simulink model "ProyectoGlobal_AyCD_Cantu_LagoTejo_OPCUA"  (R2021a)
settings: Solver=ode23  StartTime=0.0  StopTime=inf  MinStep=1e-4
undefined symbols (not defined in the file): a_hMax, a_tMax, b_cx, b_cy, b_eq_h, b_eq_t, b_hb, b_hEb, b_t, b_tb, b_tw, b_wu, bah, bat, bcx, bcy, CI_h, CI_t, Cond_Ini_h, Cond_Ini_t, g, H_c, i_h, i_t, k_cy, k_tw, k_wu, Kcy, Kd_bal, Kp_bal, ksah, ksat, ksiah, ksiat, lim_xDer, lim_xDer_ult, lim_xIzq, lim_xIzq_ult, lim_yInf, lim_yInf_ult, lim_ySup, lim_ySup_ult, M_cMax, M_cMin, M_eq_h, M_eq_t, M_s, M_t, r_hd, r_td, T_hbMax, T_hEbMax, T_hmMax, T_tbMax, T_tmMax, tau_hm, tau_tm, v_hMax_0, v_tMax, xc ... (+2)
libraries: simulink x13, opclib x3
(part 2 of 3)

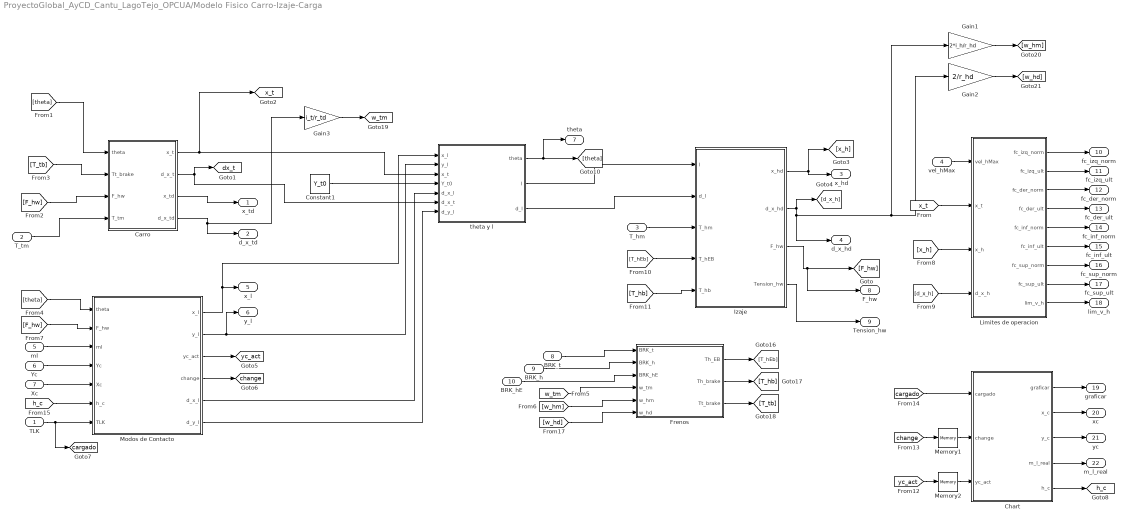
== system ProyectoGlobal_AyCD_Cantu_LagoTejo_OPCUA/Modelo Fisico Carro-Izaje-Carga ==
  TLK : Inport
  T_tm : Inport  Port=2
  T_hm : Inport  Port=3
  vel_hMax : Inport  Port=4
  ml : Inport  Port=5
  Yc : Inport  Port=6
  Xc : Inport  Port=7
  BRK_t : Inport  Port=8
  BRK_h : Inport  Port=9
  BRK_hE : Inport  Port=10
  Carro : Subsystem
  Chart : Stateflow chart  TreatAsAtomicUnit=on
      settings: PortSchema="{\"entries\":[{\"content\":{\"sides\":[{\"content\":{\"connectorIds\":[\"In1\",\"In2\",\"In3\"]},\"type\":\"ConnectorPlacement.EquallySpacedRectSide\",\"uuid\":\"3e82a7c2-bf75-4f61-8ed8-4dc94ac63b2a\"},{\"content\":{\"connectorIds\":[\"Out3\",\"Out4\",\"Out2\",\"Out5\",\"Out1\"],\"side\":\"RIGHT\"},\"type\":\"ConnectorPlacement.EquallySpacedRectSide\",\"uuid\":\"3bda0d7b-f5b8-4b7e-98a5-641e146bfa09\"},{\"content\":{\"connectorIds\":[],\"side\":\"TOP\"},\"type\":\"ConnectorPlacement.EquallySpacedRectSide\",\"uuid\":\"53c96370-adb7-4c5f-b84b-b565cd95f057\"}]},\"type\":\"ConnectorPlacement.EquallySpacedConnector\",\"uuid\":\"5926f053-77e4-4d2a-97aa-9f275575c8db\"}],\"packageUris\":[\"http://schema.mathworks.com/mf0/Connector/R2020b\"],\"version\":\"1.0\"}"
  Constant1 : Constant  Value=Y_t0
  Frenos : Subsystem
  Gain1 : Gain  Gain=2*i_h/r_hd
  Gain2 : Gain  Gain=2/r_hd
  Gain3 : Gain  Gain=i_t/r_td
  Izaje : Subsystem
  Limites de operacion : Subsystem
  Memory1 : Memory
  Memory2 : Memory
  Modos de Contacto : Subsystem
  theta y l : Subsystem
  x_td : Outport
  d_x_td : Outport  Port=2
  x_hd : Outport  Port=3
  d_x_hd : Outport  Port=4
  x_l : Outport  Port=5
  y_l : Outport  Port=6
  theta : Outport  Port=7
  F_hw : Outport  Port=8
  Tension_hw : Outport  Port=9
  fc_izq_norm : Outport  Port=10
  fc_izq_ult : Outport  Port=11
  fc_der_norm : Outport  Port=12
  fc_der_ult : Outport  Port=13
  fc_inf_norm : Outport  Port=14
  fc_inf_ult : Outport  Port=15
  fc_sup_norm : Outport  Port=16
  fc_sup_ult : Outport  Port=17
  lim_v_h : Outport  Port=18
  graficar : Outport  Port=19
  xc : Outport  Port=20
  yc : Outport  Port=21
  m_l_real : Outport  Port=22
  tag scope: cargado=global, change=global, dx_t=global, h_c=global, w_tm=global, x_t=global, yc_act=global
  wires:
  BRK_h/1 -> Frenos/2(BRK_h)
  BRK_t/1 -> Frenos/1(BRK_t)
  BRK_hE/1 -> Frenos/3(BRK_hE)
  [w_tm] -> Frenos/4(w_tm)
  [w_hm] -> Frenos/5(w_hm)
  Limites de operacion/2(fc_izq_ult) -> fc_izq_ult/1
  Limites de operacion/1(fc_izq_norm) -> fc_izq_norm/1
  Limites de operacion/6(fc_inf_ult) -> fc_inf_ult/1
  Gain2/1 -> [w_hd]
  Limites de operacion/9(lim_v_h) -> lim_v_h/1
  Limites de operacion/3(fc_der_norm) -> fc_der_norm/1
  Limites de operacion/4(fc_der_ult) -> fc_der_ult/1
  Limites de operacion/5(fc_inf_norm) -> fc_inf_norm/1
  Limites de operacion/7(fc_sup_norm) -> fc_sup_norm/1
  Gain3/1 -> [w_tm]
  vel_hMax/1 -> Limites de operacion/1(vel_hMax)
  Limites de operacion/8(fc_sup_ult) -> fc_sup_ult/1
  Gain1/1 -> [w_hm]
  Frenos/1(Th_EB) -> [T_hEb]
  Frenos/2(Th_brake) -> [T_hb]
  Frenos/3(Tt_brake) -> [T_tb]
  [w_hd] -> Frenos/6(w_hd)
  [theta] -> Carro/1(theta)
  [T_tb] -> Carro/2(Tt_brake)
  [F_hw] -> Carro/3(F_hw)
  T_tm/1 -> Carro/4(T_tm)
  Carro/2(d_x_t) -> theta y l/6(d_x_t), [dx_t]
  Carro/3(x_td) -> x_td/1
  Carro/4(d_x_td) -> Gain3/1, d_x_td/1
  Modos de Contacto/1(x_l) -> x_l/1, theta y l/1(x_l)
  Carro/1(x_t) -> [x_t], theta y l/3(x_t)
  Modos de Contacto/2(y_l) -> y_l/1, theta y l/2(y_l)
  theta y l/1(theta) -> [theta], theta/1
  Constant1/1 -> theta y l/4(Y_t0)
  Modos de Contacto/5(d_x_l) -> theta y l/5(d_x_l)
  Modos de Contacto/6(d_y_l) -> theta y l/7(d_y_l)
  [theta] -> Modos de Contacto/1(theta)
  [F_hw] -> Modos de Contacto/2(F_hw)
  ml/1 -> Modos de Contacto/3(ml)
  [h_c] -> Modos de Contacto/6(h_c)
  Yc/1 -> Modos de Contacto/4(Yc)
  Xc/1 -> Modos de Contacto/5(Xc)
  Modos de Contacto/4(change) -> [change]
  [T_hEb] -> Izaje/4(T_hEB)
  T_hm/1 -> Izaje/3(T_hm)
  [T_hb] -> Izaje/5(T_hb)
  theta y l/2(l) -> Izaje/1(l)
  theta y l/3(d_l) -> Izaje/2(d_l)
  Izaje/3(F_hw) -> F_hw/1, [F_hw]
  Izaje/1(x_hd) -> x_hd/1, [x_h]
  Izaje/2(d_x_hd) -> d_x_hd/1, Gain2/1, Gain1/1, [d_x_h]
  [x_t] -> Limites de operacion/2(x_t)
  [x_h] -> Limites de operacion/3(x_h)
  [d_x_h] -> Limites de operacion/4(d_x_h)
  Izaje/4(Tension_hw) -> Tension_hw/1
  [change] -> Memory1/1
  Chart/1(h_c) -> [h_c]
  Chart/4(x_c) -> xc/1
  Chart/3(graficar) -> graficar/1
  Chart/2(y_c) -> yc/1
  [yc_act] -> Memory2/1
  Modos de Contacto/3(yc_act) -> [yc_act]
  TLK/1 -> [cargado], Modos de Contacto/7(TLK)
  [cargado] -> Chart/1(cargado)
  Memory1/1 -> Chart/2(change)
  Memory2/1 -> Chart/3(yc_act)
  Chart/5(m_l_real) -> m_l_real/1

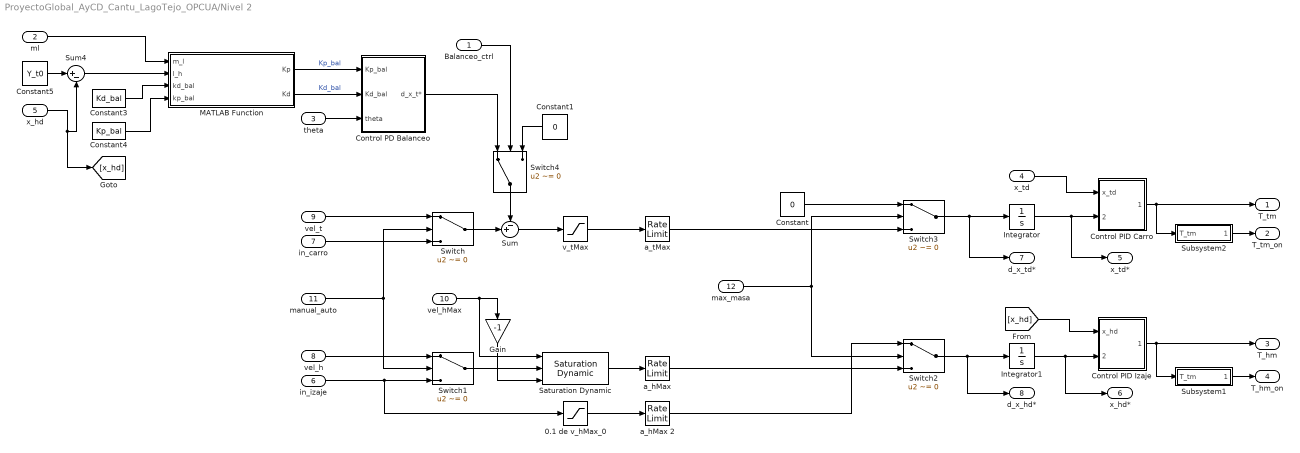
== system ProyectoGlobal_AyCD_Cantu_LagoTejo_OPCUA/Nivel 2 ==
  Balanceo_ctrl : Inport
  ml : Inport  Port=2
  theta : Inport  Port=3
  x_td : Inport  Port=4
  x_hd : Inport  Port=5
  in_izaje : Inport  Port=6
  in_carro : Inport  Port=7
  vel_h : Inport  Port=8
  vel_t : Inport  Port=9
  vel_hMax : Inport  Port=10
  manual_auto : Inport  Port=11
  max_masa : Inport  Port=12
  0.1 de v_hMax_0 : Saturate  UpperLimit=0  LowerLimit=-0.1*v_hMax_0
  Constant : Constant  Value=0
  Constant1 : Constant  Value=0
  Constant3 : Constant  Value=Kd_bal
  Constant4 : Constant  Value=Kp_bal
  Constant5 : Constant  Value=Y_t0
  Control PD Balanceo : Subsystem
  Control PID Carro : Subsystem
  Control PID Izaje : Subsystem
  Gain : Gain  Gain=-1
  Integrator : Integrator  InitialCondition=CI_t
  Integrator1 : Integrator  InitialCondition=CI_h
  MATLAB Function : MATLAB Function  TreatAsAtomicUnit=on
  Saturation Dynamic : simulink/Discontinuities/Saturation Dynamic  OutMin=[]  OutMax=[]  OutDataTypeStr=Inherit: Same as second input  OutDataType=fixdt(1, 16)  OutScaling=2^-10  DoSatur=off
  Subsystem1 : Subsystem
  Subsystem2 : Subsystem
  Sum : Sum  Inputs=-+|
  Sum4 : Sum  Inputs=|+-
  Switch{,1..4} (5 alike) : Switch  Criteria=u2 ~= 0
  a_hMax : RateLimiter  RisingSlewLimit=a_hMax  FallingSlewLimit=-a_hMax  SampleTimeMode=inherited
  a_hMax 2 : RateLimiter  RisingSlewLimit=a_hMax  FallingSlewLimit=-a_hMax  SampleTimeMode=inherited
  a_tMax : RateLimiter  RisingSlewLimit=a_tMax  FallingSlewLimit=-a_tMax  SampleTimeMode=inherited
  v_tMax : Saturate  UpperLimit=v_tMax  LowerLimit=-v_tMax
  T_tm : Outport
  T_tm_on : Outport  Port=2
  T_hm : Outport  Port=3
  T_hm_on : Outport  Port=4
  x_td* : Outport  Port=5
  x_hd* : Outport  Port=6
  d_x_td* : Outport  Port=7
  d_x_hd* : Outport  Port=8
  wires:
  manual_auto/1 -> Switch/2, Switch1/2
  Switch1/1 -> Saturation Dynamic/2
  vel_hMax/1 -> Saturation Dynamic/1, Gain/1
  Gain/1 -> Saturation Dynamic/3
  in_carro/1 -> Switch/3
  vel_h/1 -> Switch1/1
  Saturation Dynamic/1 -> a_hMax/1
  v_tMax/1 -> a_tMax/1
  Constant/1 -> Switch3/1
  0.1 de v_hMax_0/1 -> a_hMax 2/1
  vel_t/1 -> Switch/1
  Switch/1 -> Sum/2
  in_izaje/1 -> 0.1 de v_hMax_0/1, Switch1/3
  max_masa/1 -> Switch2/2, Switch3/2
  a_hMax 2/1 -> Switch2/1
  Sum/1 -> v_tMax/1
  a_tMax/1 -> Switch3/3
  a_hMax/1 -> Switch2/3
  Constant3/1 -> MATLAB Function/3(kd_bal)
  Balanceo_ctrl/1 -> Switch4/2
  Constant4/1 -> MATLAB Function/4(kp_bal)
  Constant5/1 -> Sum4/1
  x_hd/1 -> [x_hd], Sum4/2
  Sum4/1 -> MATLAB Function/2(l_h)
  ml/1 -> MATLAB Function/1(m_l)
  Constant1/1 -> Switch4/3
  MATLAB Function/1(Kp) -> Control PD Balanceo/1(Kp_bal)  "Kp_bal"
  MATLAB Function/2(Kd) -> Control PD Balanceo/2(Kd_bal)  "Kd_bal"
  theta/1 -> Control PD Balanceo/3(theta)
  Control PD Balanceo/1(d_x_t*) -> Switch4/1
  Switch4/1 -> Sum/1
  x_td/1 -> Control PID Carro/1(x_td)
  Integrator1/1 -> x_hd*/1, Control PID Izaje/2(x_hd*)
  [x_hd] -> Control PID Izaje/1(x_hd)
  Switch2/1 -> d_x_hd*/1, Integrator1/1
  Control PID Carro/1(T_tm) -> Subsystem2/1(T_tm), T_tm/1
  Integrator/1 -> x_td*/1, Control PID Carro/2(x_td*)
  Switch3/1 -> d_x_td*/1, Integrator/1
  Control PID Izaje/1(T_hm) -> T_hm/1, Subsystem1/1(T_tm)
  Subsystem1/1(T_tm_on) -> T_hm_on/1
  Subsystem2/1(T_tm_on) -> T_tm_on/1

== system ProyectoGlobal_AyCD_Cantu_LagoTejo_OPCUA/Subsystem ==
  " " : Inport
  AND : Logic  IconShape=distinctive  AllPortsSameDT=off  OutDataTypeStr=boolean
  BTN_RESET_PRESSED : Constant  Value=0
  Out1 : Outport
  wires:
  BTN_RESET_PRESSED/1 -> AND/2
  " "/1 -> AND/1
  AND/1 -> Out1/1

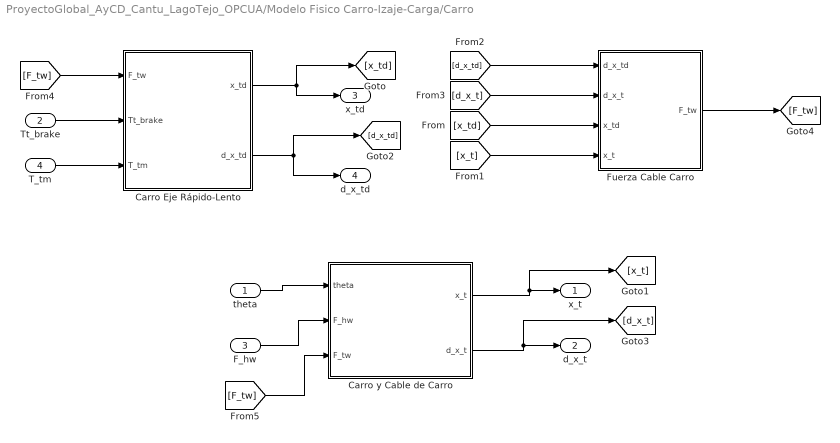
== system ProyectoGlobal_AyCD_Cantu_LagoTejo_OPCUA/Modelo Fisico Carro-Izaje-Carga/Carro ==
  theta : Inport
  Tt_brake : Inport  Port=2
  F_hw : Inport  Port=3
  T_tm : Inport  Port=4
  Carro Eje Rápido-Lento : Subsystem
  Carro y Cable de Carro : Subsystem
  Fuerza Cable Carro : Subsystem
  x_t : Outport
  d_x_t : Outport  Port=2
  x_td : Outport  Port=3
  d_x_td : Outport  Port=4
  wires:
  Tt_brake/1 -> Carro Eje Rápido-Lento/2(Tt_brake)
  theta/1 -> Carro y Cable de Carro/1(theta)
  Carro Eje Rápido-Lento/1(x_td) -> x_td/1, [x_td]
  Carro y Cable de Carro/2(d_x_t) -> [d_x_t], d_x_t/1
  Carro Eje Rápido-Lento/2(d_x_td) -> [d_x_td], d_x_td/1
  F_hw/1 -> Carro y Cable de Carro/2(F_hw)
  Carro y Cable de Carro/1(x_t) -> [x_t], x_t/1
  T_tm/1 -> Carro Eje Rápido-Lento/3(T_tm)
  [x_td] -> Fuerza Cable Carro/3(x_td)
  [x_t] -> Fuerza Cable Carro/4(x_t)
  Fuerza Cable Carro/1(F_tw) -> [F_tw]
  [d_x_td] -> Fuerza Cable Carro/1(d_x_td)
  [d_x_t] -> Fuerza Cable Carro/2(d_x_t)
  [F_tw] -> Carro Eje Rápido-Lento/1(F_tw)
  [F_tw] -> Carro y Cable de Carro/3(F_tw)

== system ProyectoGlobal_AyCD_Cantu_LagoTejo_OPCUA/Modelo Fisico Carro-Izaje-Carga/Frenos ==
  BRK_t : Inport
  BRK_h : Inport  Port=2
  BRK_hE : Inport  Port=3
  w_tm : Inport  Port=4
  w_hm : Inport  Port=5
  w_hd : Inport  Port=6
  Freno Emergencia Izaje : Subsystem
  Freno Operacion Carro : Subsystem
  Freno Operacion Izaje : Subsystem
  Th_EB : Outport
  Th_brake : Outport  Port=2
  Tt_brake : Outport  Port=3
  wires:
  Freno Operacion Izaje/1(Thb) -> Th_brake/1
  BRK_h/1 -> Freno Operacion Izaje/1(Energizado/Desenergizado)
  BRK_t/1 -> Freno Operacion Carro/1(Energizado/Desenergizado)
  Freno Operacion Carro/1(Ttb) -> Tt_brake/1
  BRK_hE/1 -> Freno Emergencia Izaje/1(Energizado/Desenergizado)
  Freno Emergencia Izaje/1(Th_EB) -> Th_EB/1
  w_tm/1 -> Freno Operacion Carro/2(w_tm)
  w_hm/1 -> Freno Operacion Izaje/2(w_hm)
  w_hd/1 -> Freno Emergencia Izaje/2(w_hd)

== system ProyectoGlobal_AyCD_Cantu_LagoTejo_OPCUA/Modelo Fisico Carro-Izaje-Carga/Izaje ==
  l : Inport
  d_l : Inport  Port=2
  T_hm : Inport  Port=3
  T_hEB : Inport  Port=4
  T_hb : Inport  Port=5
  Fuerza cable de Izaje : Subsystem
  Izaje Eje Rapido-Lento : Subsystem
  x_hd : Outport
  d_x_hd : Outport  Port=2
  F_hw : Outport  Port=3
  Tension_hw : Outport  Port=4
  wires:
  T_hb/1 -> Izaje Eje Rapido-Lento/4(T_hb)
  T_hEB/1 -> Izaje Eje Rapido-Lento/3(T_hEb)
  [F_hw] -> Izaje Eje Rapido-Lento/1(F_hw)
  T_hm/1 -> Izaje Eje Rapido-Lento/2(T_hm)
  Fuerza cable de Izaje/1(F_hw) -> [F_hw], F_hw/1
  d_l/1 -> Fuerza cable de Izaje/3(d_l)
  Izaje Eje Rapido-Lento/1(l_h) -> [l_h]
  Izaje Eje Rapido-Lento/3(x_hd) -> x_hd/1
  l/1 -> Fuerza cable de Izaje/1(l)
  Izaje Eje Rapido-Lento/4(d_x_hd) -> d_x_hd/1
  [l_h] -> Fuerza cable de Izaje/2(l_h)
  Izaje Eje Rapido-Lento/2(d_l_h) -> [d_l_h]
  [d_l_h] -> Fuerza cable de Izaje/4(d_l_h)
  Fuerza cable de Izaje/2(Tension_hw) -> Tension_hw/1

== system ProyectoGlobal_AyCD_Cantu_LagoTejo_OPCUA/Modelo Fisico Carro-Izaje-Carga/Limites de operacion ==
  vel_hMax : Inport
  x_t : Inport  Port=2
  x_h : Inport  Port=3
  d_x_h : Inport  Port=4
  Límites de Carro : Subsystem
  Subsystem1 : Subsystem
  fc_izq_norm : Outport
  fc_izq_ult : Outport  Port=2
  fc_der_norm : Outport  Port=3
  fc_der_ult : Outport  Port=4
  fc_inf_norm : Outport  Port=5
  fc_inf_ult : Outport  Port=6
  fc_sup_norm : Outport  Port=7
  fc_sup_ult : Outport  Port=8
  lim_v_h : Outport  Port=9
  wires:
  x_t/1 -> Límites de Carro/1(x_t)
  Límites de Carro/1(fc_izq_norm) -> fc_izq_norm/1
  Límites de Carro/2(fc_izq_ult) -> fc_izq_ult/1
  Límites de Carro/3(fc_der_norm) -> fc_der_norm/1
  Límites de Carro/4(fc_der_ult) -> fc_der_ult/1
  Subsystem1/4(fc_sup_ult) -> fc_sup_ult/1
  Subsystem1/3(fc_sup_norm) -> fc_sup_norm/1
  Subsystem1/2(fc_inf_ult) -> fc_inf_ult/1
  Subsystem1/1(fc_inf_norm) -> fc_inf_norm/1
  x_h/1 -> Subsystem1/1(x_h)
  d_x_h/1 -> Subsystem1/3(d_x_h)
  Subsystem1/5(lim_v_h) -> lim_v_h/1
  vel_hMax/1 -> Subsystem1/2(vel_hMax)

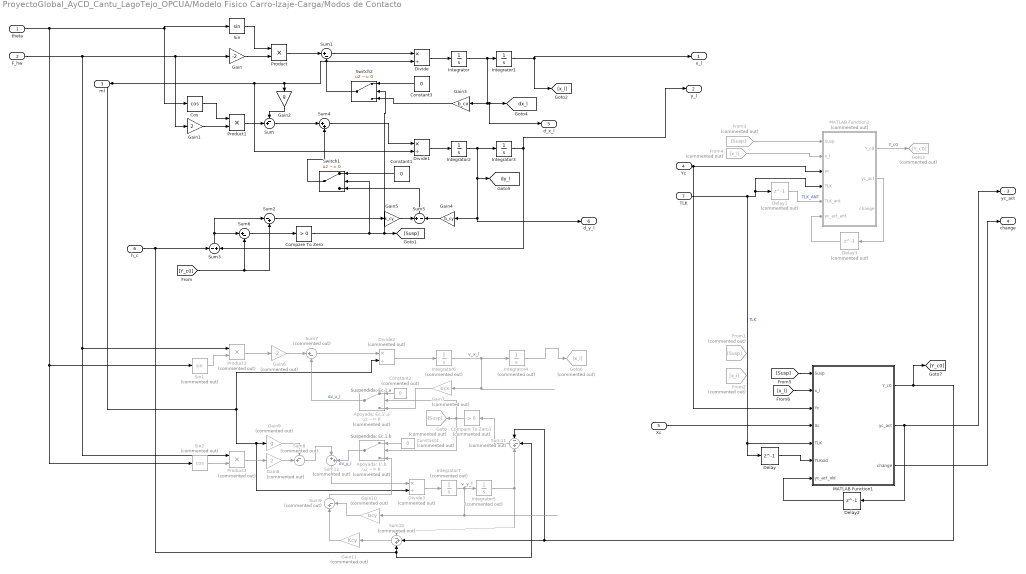
== system ProyectoGlobal_AyCD_Cantu_LagoTejo_OPCUA/Modelo Fisico Carro-Izaje-Carga/Modos de Contacto ==
  note: v_y_l
  note: v_x_l
  note: Suspendida: Ec.1.a
  note: Suspendida: Ec.1.b
  theta : Inport
  F_hw : Inport  Port=2
  ml : Inport  Port=3
  Yc : Inport  Port=4
  Xc : Inport  Port=5
  h_c : Inport  Port=6
  TLK : Inport  Port=7
  Apoyada: 1'.b : Switch  Commented=on  Criteria=u2 ~= 0
  Apoyada: Ec.1'.a : Switch  Commented=on  Criteria=u2 ~= 0
  Compare To Zero : simulink/Logic and Bit Operations/Compare To Zero  relop=>  OutDataTypeStr=boolean
  Compare To Zero1 : simulink/Logic and Bit Operations/Compare To Zero  Commented=on  relop=>  OutDataTypeStr=boolean
  Constant1 : Constant  Value=0
  Constant2 : Constant  Commented=on  Value=0
  Constant3 : Constant  Value=0
  Constant4 : Constant  Commented=on  Value=0
  Cos : Trigonometry  Operator=cos
  Delay : Delay  DelayLength=1
  Delay1 : Delay  Commented=on  DelayLength=1
  Delay2 : Delay  DelayLength=1
  Delay3 : Delay  Commented=on  DelayLength=1
  Divide : Product  Inputs=*/
  Divide1 : Product  Inputs=*/
  Divide2 : Product  Commented=on  Inputs=*/
  Divide3 : Product  Commented=on  Inputs=*/
  From1 : From  Commented=on  GotoTag=Susp
  From2 : From  Commented=on  GotoTag=x_l
  From3 : From  Commented=on  GotoTag=Susp
  From4 : From  Commented=on  GotoTag=x_l
  Gain : Gain  Gain=-2
  Gain1 : Gain  Gain=2
  Gain10 : Gain  Commented=on  Gain=bcy
  Gain11 : Gain  Commented=on  Gain=Kcy
  Gain2 : Gain  Gain=g
  Gain3 : Gain  Gain=b_cx
  Gain4 : Gain  Gain=b_cy
  Gain5 : Gain  Gain=k_cy
  Gain6 : Gain  Commented=on  Gain=-2
  Gain7 : Gain  Commented=on  Gain=bcx
  Gain8 : Gain  Commented=on  Gain=2
  Gain9 : Gain  Commented=on  Gain=g
  Goto : Goto  Commented=on  GotoTag=Susp
  Goto3 : Goto  Commented=on  GotoTag=Y_c0
  Goto6 : Goto  Commented=on  GotoTag=x_l
  Integrator : Integrator
  Integrator1 : Integrator  InitialCondition=CI_t
  Integrator2 : Integrator
  Integrator3 : Integrator  InitialCondition=CI_h
  Integrator4 : Integrator  Commented=on  InitialCondition=Cond_Ini_t
  Integrator5 : Integrator  Commented=on  InitialCondition=Cond_Ini_h
  Integrator6 : Integrator  Commented=on
  Integrator7 : Integrator  Commented=on
  MATLAB Function1 : MATLAB Function  TreatAsAtomicUnit=on
  MATLAB Function2 : MATLAB Function  Commented=on  TreatAsAtomicUnit=on
  Product : Product
  Product1 : Product
  Product2 : Product  Commented=on
  Product3 : Product  Commented=on
  Sin : Trigonometry
  Sin1 : Trigonometry  Commented=on
  Sin2 : Trigonometry  Commented=on  Operator=cos
  Sum : Sum  Inputs=-+|
  Sum1 : Sum  Inputs=|+-
  Sum10 : Sum  Commented=on  Inputs=-++
  Sum11 : Sum  Commented=on  Inputs=--+
  Sum12 : Sum  Commented=on  Inputs=|++
  Sum2 : Sum  Inputs=|-+
  Sum3 : Sum  Inputs=-|+
  Sum4 : Sum  Inputs=|++
  Sum5 : Sum  Inputs=+|-
  Sum6 : Sum  Inputs=|+-
  Sum7 : Sum  Commented=on  Inputs=|+-
  Sum8 : Sum  Commented=on  Inputs=-+|
  Sum9 : Sum  Commented=on  Inputs=|+-
  Switch1 : Switch  Criteria=u2 ~= 0
  Switch2 : Switch  Criteria=u2 ~= 0
  x_l : Outport
  y_l : Outport  Port=2
  yc_act : Outport  Port=3
  change : Outport  Port=4
  d_x_l : Outport  Port=5
  d_y_l : Outport  Port=6
  tag scope: dx_l=global, dy_l=global
  wires:
  Gain/1 -> Product/2
  Sin/1 -> Product/1
  Cos/1 -> Product1/1
  Gain1/1 -> Product1/2
  Divide/1 -> Integrator/1
  Integrator/1 -> Integrator1/1, d_x_l/1, [dx_l], Gain3/1
  Divide1/1 -> Integrator2/1
  Integrator2/1 -> [dy_l], d_y_l/1, Gain4/1, Integrator3/1
  Integrator3/1 -> Sum3/2, y_l/1
  Product/1 -> Sum1/1
  Sum1/1 -> Divide/1
  Switch2/1 -> Sum1/2
  Constant3/1 -> Switch2/1
  Gain3/1 -> Switch2/3
  Sum5/1 -> Switch1/3
  Gain5/1 -> Sum5/1
  Gain4/1 -> Sum5/2
  Constant1/1 -> Switch1/1
  h_c/1 -> Sum3/1, Sum11/2, Sum10/3
  Sum3/1 -> Sum6/1, Sum2/1
  Sum/1 -> Sum4/1
  Sum4/1 -> Divide1/1
  Switch1/1 -> Sum4/2
  Product1/1 -> Sum/2
  Gain2/1 -> Sum/1
  Integrator1/1 -> [x_l], x_l/1
  Sum2/1 -> Gain5/1
  Sum6/1 -> Compare To Zero/1
  F_hw/1 -> Product3/1, Product2/1, Gain/1, Gain1/1
  Compare To Zero/1 -> [Susp], Switch2/2, Switch1/2
  From4/1 -> MATLAB Function2/2(x_l)
  MATLAB Function2/1(Y_c0) -> Goto3/1  "Y_c0"
  MATLAB Function2/2(yc_act) -> Delay3/1
  From3/1 -> MATLAB Function2/1(Susp)
  Delay1/1 -> MATLAB Function2/5(TLK_ant)  "TLK_ANT"
  TLK/1 -> Delay/1, MATLAB Function1/5(TLK), MATLAB Function2/4(TLK), Delay1/1  "TLK"
  Delay3/1 -> MATLAB Function2/6(yc_act_ant)
  Sum8/1 -> Sum12/1
  Constant2/1 -> Apoyada: Ec.1'.a/1
  Divide3/1 -> Integrator7/1
  Gain6/1 -> Sum7/1
  Sin2/1 -> Product3/2
  Yc/1 -> MATLAB Function2/3(yc), MATLAB Function1/3(Yc)
  Xc/1 -> MATLAB Function1/4(Xc)
  Sum7/1 -> Divide2/1
  ml/1 -> Divide/2, Gain2/1, Divide1/2, Divide2/2, Divide3/2, Gain9/1
  MATLAB Function1/2(yc_act) -> yc_act/1, Delay2/1
  MATLAB Function1/3(change) -> change/1
  Delay2/1 -> MATLAB Function1/7(yc_act_old)
  Sin1/1 -> Product2/2
  [x_l] -> MATLAB Function1/2(x_l)
  [Susp] -> MATLAB Function1/1(Susp)
  MATLAB Function1/1(Y_c0) -> [Y_c0], Sum10/2, Sum11/1
  Delay/1 -> MATLAB Function1/6(TLKold)
  Sum11/1 -> Compare To Zero1/1
  Sum10/1 -> Gain11/1
  Integrator6/1 -> Gain7/1, Integrator4/1
  Gain8/1 -> Sum8/2
  Gain9/1 -> Sum8/1
  Product2/1 -> Gain6/1
  Product3/1 -> Gain8/1
  Apoyada: Ec.1'.a/1 -> Sum7/2  "dv_x_l"
  Divide2/1 -> Integrator6/1
  theta/1 -> Sin2/1, Sin1/1, Sin/1, Cos/1
  Sum12/1 -> Divide3/1
  Compare To Zero1/1 -> Goto/1, Apoyada: Ec.1'.a/2, Apoyada: 1'.b/2
  Sum9/1 -> Apoyada: 1'.b/3
  Gain7/1 -> Apoyada: Ec.1'.a/3
  Gain10/1 -> Sum9/2
  Gain11/1 -> Sum9/1
  Integrator7/1 -> Gain10/1, Integrator5/1
  Constant4/1 -> Apoyada: 1'.b/1
  Integrator5/1 -> Sum11/3, Sum10/1
  Apoyada: 1'.b/1 -> Sum12/2  "dv_y_l"
  Integrator4/1 -> Goto6/1
  [Y_c0] -> Sum2/2, Sum6/2

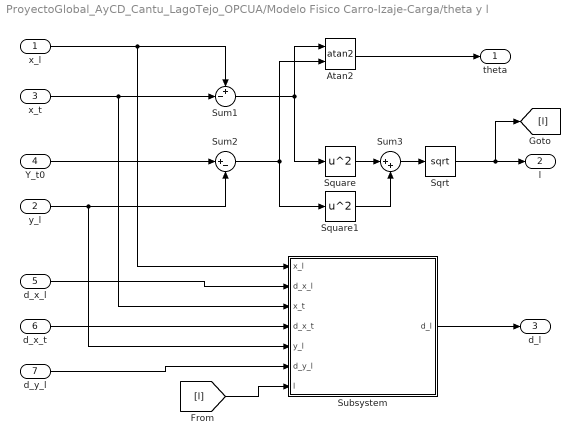
== system ProyectoGlobal_AyCD_Cantu_LagoTejo_OPCUA/Modelo Fisico Carro-Izaje-Carga/theta y l ==
  x_l : Inport
  y_l : Inport  Port=2
  x_t : Inport  Port=3
  Y_t0 : Inport  Port=4
  d_x_l : Inport  Port=5
  d_x_t : Inport  Port=6
  d_y_l : Inport  Port=7
  Atan2 : Trigonometry  Operator=atan2
  Sqrt : Sqrt  SaturateOnIntegerOverflow=on
  Square : Math  Operator=square  SaturateOnIntegerOverflow=on
  Square1 : Math  Operator=square  SaturateOnIntegerOverflow=on
  Subsystem : Subsystem
  Sum1 : Sum  Inputs=+-|
  Sum2 : Sum  Inputs=|+-
  Sum3 : Sum  Inputs=|++
  theta : Outport
  l : Outport  Port=2
  d_l : Outport  Port=3
  wires:
  x_l/1 -> Subsystem/1(x_l), Sum1/1
  x_t/1 -> Subsystem/3(x_t), Sum1/2
  Y_t0/1 -> Sum2/1
  y_l/1 -> Subsystem/5(y_l), Sum2/2
  Sum1/1 -> Square/1, Atan2/1
  Sum2/1 -> Square1/1, Atan2/2
  Sum3/1 -> Sqrt/1
  Sqrt/1 -> [l], l/1
  Square/1 -> Sum3/1
  Square1/1 -> Sum3/2
  Atan2/1 -> theta/1
  [l] -> Subsystem/7(l)
  d_x_l/1 -> Subsystem/2(d_x_l)
  d_x_t/1 -> Subsystem/4(d_x_t)
  d_y_l/1 -> Subsystem/6(d_y_l)
  Subsystem/1(d_l) -> d_l/1

== system ProyectoGlobal_AyCD_Cantu_LagoTejo_OPCUA/Nivel 2/Control PD Balanceo ==
  Kp_bal : Inport
  Kd_bal : Inport  Port=2
  theta : Inport  Port=3
  Constant2 : Constant  Value=0
  Delay One Step : Delay  DelayLength=1  SampleTime=1e-3
  Gain1 : Gain  Gain=1/1e-3
  Product : Product
  Product1 : Product
  Sum1 : Sum  Inputs=|+-
  Sum2 : Sum  Inputs=|+-
  Sum3 : Sum  Inputs=|++
  d_x_t* : Outport
  wires:
  Product1/1 -> Sum3/1
  Gain1/1 -> Product/2
  Kp_bal/1 -> Product1/1
  Product/1 -> Sum3/2
  Sum2/1 -> Gain1/1
  Constant2/1 -> Sum1/1
  Sum1/1 -> Product1/2, Sum2/1, Delay One Step/1
  Delay One Step/1 -> Sum2/2
  theta/1 -> Sum1/2
  Kd_bal/1 -> Product/1
  Sum3/1 -> d_x_t*/1

== system ProyectoGlobal_AyCD_Cantu_LagoTejo_OPCUA/Nivel 2/Control PID Carro ==
  x_td : Inport
  x_td* : Inport  Port=2
  Gain : Gain  Gain=1/tau_tm
  Integrator : Integrator  InitialConditionSource=external
  PID Traslacion : Subsystem
  Sum : Sum  Inputs=|+-
  T_tmMax : Saturate  UpperLimit=T_tmMax  LowerLimit=-T_tmMax
  T_tm : Outport
  wires:
  PID Traslacion/1(T_tm*) -> T_tmMax/1
  x_td*/1 -> PID Traslacion/1(x_td*)
  x_td/1 -> PID Traslacion/2(x_td)
  T_tmMax/1 -> Integrator/2, Sum/1
  Sum/1 -> Gain/1
  Gain/1 -> Integrator/1
  Integrator/1 -> T_tm/1, Sum/2

== system ProyectoGlobal_AyCD_Cantu_LagoTejo_OPCUA/Nivel 2/Control PID Izaje ==
  x_hd : Inport
  x_hd* : Inport  Port=2
  Gain : Gain  Gain=1/tau_hm
  Integrator : Integrator  InitialConditionSource=external
  PID Izaje : Subsystem
  Saturation1 : Saturate  UpperLimit=T_hmMax  LowerLimit=-T_hmMax
  Sum : Sum  Inputs=|+-
  T_hm : Outport
  wires:
  PID Izaje/1(T_hm) -> Saturation1/1
  x_hd*/1 -> PID Izaje/1(x_h*)
  x_hd/1 -> PID Izaje/2(x_h)
  Gain/1 -> Integrator/1
  Sum/1 -> Gain/1
  Saturation1/1 -> Integrator/2, Sum/1
  Integrator/1 -> T_hm/1, Sum/2

== system ProyectoGlobal_AyCD_Cantu_LagoTejo_OPCUA/Nivel 2/Subsystem1 ==
  T_tm : Inport
  AND : Logic  Operator=NAND  Inputs=3  IconShape=distinctive  AllPortsSameDT=off  OutDataTypeStr=boolean
  Abs1 : Abs
  Abs2 : Abs
  Abs3 : Abs
  Compare To Constant1 : simulink/Logic and Bit Operations/Compare To Constant  relop=<  const=1e-3  OutDataTypeStr=boolean
  Compare To Constant2 : simulink/Logic and Bit Operations/Compare To Constant  relop=<  const=1e-3  OutDataTypeStr=boolean
  Compare To Constant3 : simulink/Logic and Bit Operations/Compare To Constant  relop=<  const=1e-3  OutDataTypeStr=boolean
  Memory : Memory
  Memory1 : Memory
  T_tm_on : Outport
  wires:
  Abs1/1 -> Compare To Constant1/1
  T_tm/1 -> Abs1/1, Memory/1
  Abs2/1 -> Compare To Constant2/1
  Memory/1 -> Abs2/1, Memory1/1
  Abs3/1 -> Compare To Constant3/1
  Memory1/1 -> Abs3/1
  Compare To Constant1/1 -> AND/1
  Compare To Constant2/1 -> AND/2
  Compare To Constant3/1 -> AND/3
  AND/1 -> T_tm_on/1

== system ProyectoGlobal_AyCD_Cantu_LagoTejo_OPCUA/Nivel 2/Subsystem2 ==
  T_tm : Inport
  AND : Logic  Operator=NAND  Inputs=3  IconShape=distinctive  AllPortsSameDT=off  OutDataTypeStr=boolean
  Abs1 : Abs
  Abs2 : Abs
  Abs3 : Abs
  Compare To Constant1 : simulink/Logic and Bit Operations/Compare To Constant  relop=<  const=1e-3  OutDataTypeStr=boolean
  Compare To Constant2 : simulink/Logic and Bit Operations/Compare To Constant  relop=<  const=1e-3  OutDataTypeStr=boolean
  Compare To Constant3 : simulink/Logic and Bit Operations/Compare To Constant  relop=<  const=1e-3  OutDataTypeStr=boolean
  Memory : Memory
  Memory1 : Memory
  T_tm_on : Outport
  wires:
  Abs1/1 -> Compare To Constant1/1
  T_tm/1 -> Abs1/1, Memory/1
  Abs2/1 -> Compare To Constant2/1
  Memory/1 -> Abs2/1, Memory1/1
  Abs3/1 -> Compare To Constant3/1
  Memory1/1 -> Abs3/1
  Compare To Constant1/1 -> AND/1
  Compare To Constant2/1 -> AND/2
  Compare To Constant3/1 -> AND/3
  AND/1 -> T_tm_on/1

== system ProyectoGlobal_AyCD_Cantu_LagoTejo_OPCUA/Modelo Fisico Carro-Izaje-Carga/Carro/Carro Eje Rápido-Lento ==
  F_tw : Inport
  Tt_brake : Inport  Port=2
  T_tm : Inport  Port=3
  1/Meq_t : Gain  Gain=1/M_eq_t
  Gain3 : Gain  Gain=i_t/r_td
  Integrator2 : Integrator
  Integrator3 : Integrator  InitialCondition=CI_t
  Sum : Sum  Inputs=|++
  Sum1 : Sum  Inputs=-+-
  beq_t : Gain  Gain=b_eq_t
  x_td : Outport
  d_x_td : Outport  Port=2
  wires:
  Integrator2/1 -> d_x_td/1, beq_t/1, Integrator3/1
  Integrator3/1 -> x_td/1
  1/Meq_t/1 -> Integrator2/1
  Sum1/1 -> 1/Meq_t/1
  beq_t/1 -> Sum1/3
  F_tw/1 -> Sum1/1
  T_tm/1 -> Sum/1  "Tmotor"
  Tt_brake/1 -> Sum/2  "Tt_brake"
  Sum/1 -> Gain3/1
  Gain3/1 -> Sum1/2

== system ProyectoGlobal_AyCD_Cantu_LagoTejo_OPCUA/Modelo Fisico Carro-Izaje-Carga/Carro/Carro y Cable de Carro ==
  theta : Inport
  F_hw : Inport  Port=2
  F_tw : Inport  Port=3
  1/M_t : Gain  Gain=1/M_t
  Gain : Gain  Gain=2
  Integrator : Integrator  InitialCondition=CI_t
  Integrator2 : Integrator
  Product : Product
  Sin : Trigonometry
  Sum1 : Sum  Inputs=++-
  b_t : Gain  Gain=b_t
  x_t : Outport
  d_x_t : Outport  Port=2
  wires:
  Sum1/1 -> 1/M_t/1
  Integrator2/1 -> d_x_t/1, b_t/1, Integrator/1
  theta/1 -> Sin/1
  Sin/1 -> Product/2
  F_hw/1 -> Gain/1
  Gain/1 -> Product/1
  Product/1 -> Sum1/2
  b_t/1 -> Sum1/3
  1/M_t/1 -> Integrator2/1
  Integrator/1 -> x_t/1
  F_tw/1 -> Sum1/1

== system ProyectoGlobal_AyCD_Cantu_LagoTejo_OPCUA/Modelo Fisico Carro-Izaje-Carga/Carro/Fuerza Cable Carro ==
  d_x_td : Inport
  d_x_t : Inport  Port=2
  x_td : Inport  Port=3
  x_t : Inport  Port=4
  Gain : Gain  Gain=k_tw
  Gain1 : Gain  Gain=b_tw
  Sum : Sum  Inputs=+|-
  Sum1 : Sum  Inputs=+|-
  Sum2 : Sum  Inputs=+|+
  F_tw : Outport
  wires:
  x_td/1 -> Sum/1
  Gain/1 -> Sum2/2
  Gain1/1 -> Sum2/1
  d_x_td/1 -> Sum1/1
  x_t/1 -> Sum/2
  Sum1/1 -> Gain1/1
  Sum2/1 -> F_tw/1
  Sum/1 -> Gain/1
  d_x_t/1 -> Sum1/2

== system ProyectoGlobal_AyCD_Cantu_LagoTejo_OPCUA/Modelo Fisico Carro-Izaje-Carga/Frenos/Freno Emergencia Izaje ==
  Energizado/Desenergizado : Inport
  w_hd : Inport  Port=2
  Constant : Constant  Value=0
  Gain : Gain  Gain=-b_hEb
  Saturation : Saturate  UpperLimit=T_hEbMax  LowerLimit=-T_hEbMax
  Switch : Switch  Criteria=u2 ~= 0
  Th_EB : Outport
  wires:
  Energizado/Desenergizado/1 -> Switch/2
  Constant/1 -> Switch/1
  w_hd/1 -> Gain/1
  Gain/1 -> Saturation/1
  Saturation/1 -> Switch/3
  Switch/1 -> Th_EB/1

== system ProyectoGlobal_AyCD_Cantu_LagoTejo_OPCUA/Modelo Fisico Carro-Izaje-Carga/Frenos/Freno Operacion Carro ==
  Energizado/Desenergizado : Inport
  w_tm : Inport  Port=2
  Constant : Constant  Value=0
  Gain : Gain  Gain=-b_tb
  Saturation : Saturate  UpperLimit=T_tbMax  LowerLimit=-T_tbMax
  Switch : Switch  Criteria=u2 ~= 0
  Ttb : Outport
  wires:
  Energizado/Desenergizado/1 -> Switch/2
  Constant/1 -> Switch/1
  w_tm/1 -> Gain/1
  Gain/1 -> Saturation/1
  Saturation/1 -> Switch/3
  Switch/1 -> Ttb/1

== system ProyectoGlobal_AyCD_Cantu_LagoTejo_OPCUA/Modelo Fisico Carro-Izaje-Carga/Frenos/Freno Operacion Izaje ==
  Energizado/Desenergizado : Inport
  w_hm : Inport  Port=2
  Constant : Constant  Value=0
  Gain : Gain  Gain=-b_hb
  Saturation : Saturate  UpperLimit=T_hbMax  LowerLimit=-T_hbMax
  Switch : Switch  Criteria=u2 ~= 0
  Thb : Outport
  wires:
  Energizado/Desenergizado/1 -> Switch/2
  Constant/1 -> Switch/1
  w_hm/1 -> Gain/1
  Gain/1 -> Saturation/1
  Saturation/1 -> Switch/3
  Switch/1 -> Thb/1

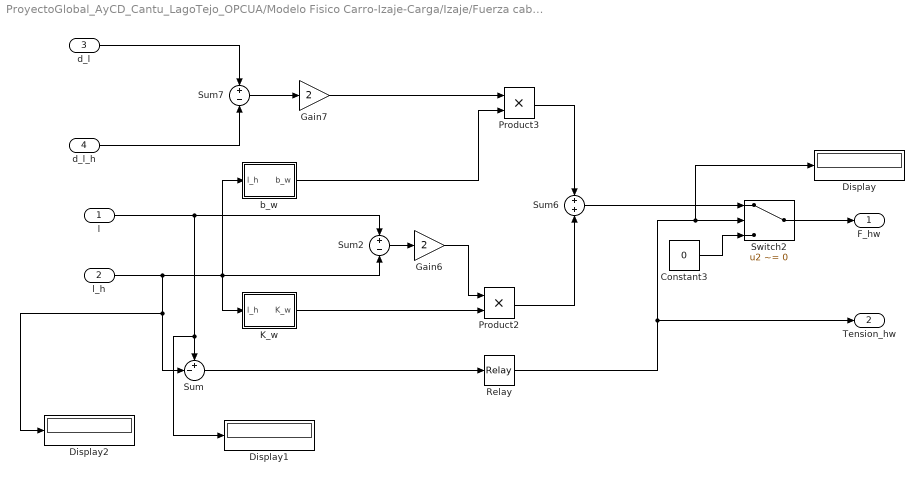
== system ProyectoGlobal_AyCD_Cantu_LagoTejo_OPCUA/Modelo Fisico Carro-Izaje-Carga/Izaje/Fuerza cable de Izaje ==
  l : Inport
  l_h : Inport  Port=2
  d_l : Inport  Port=3
  d_l_h : Inport  Port=4
  Constant3 : Constant  Value=0  SampleTime=-1
  Display : Display
  Display1 : Display
  Display2 : Display
  Gain6 : Gain  Gain=2
  Gain7 : Gain  Gain=2
  K_w : Subsystem
  Product2 : Product
  Product3 : Product
  Relay : Relay  OnSwitchValue=1e-4  OffSwitchValue=-1e-9
  Sum : Sum  Inputs=+-|
  Sum2 : Sum  Inputs=+|-
  Sum6 : Sum  Inputs=+|+
  Sum7 : Sum  Inputs=+|-
  Switch2 : Switch  Criteria=u2 ~= 0  RndMeth=Nearest  ZeroCross=off
  b_w : Subsystem
  F_hw : Outport
  Tension_hw : Outport  Port=2
  wires:
  Sum2/1 -> Gain6/1
  Constant3/1 -> Switch2/3
  l_h/1 -> Display2/1, Sum/2, K_w/1(l_h), b_w/1(l_h), Sum2/2
  Gain6/1 -> Product2/1
  K_w/1(K_w) -> Product2/2
  Sum7/1 -> Gain7/1
  Gain7/1 -> Product3/1
  b_w/1(b_w) -> Product3/2
  Product2/1 -> Sum6/2
  Product3/1 -> Sum6/1
  Sum6/1 -> Switch2/1
  l/1 -> Sum2/1, Display1/1, Sum/1
  Sum/1 -> Relay/1
  Switch2/1 -> F_hw/1
  d_l_h/1 -> Sum7/2
  d_l/1 -> Sum7/1
  Relay/1 -> Display/1, Switch2/2, Tension_hw/1

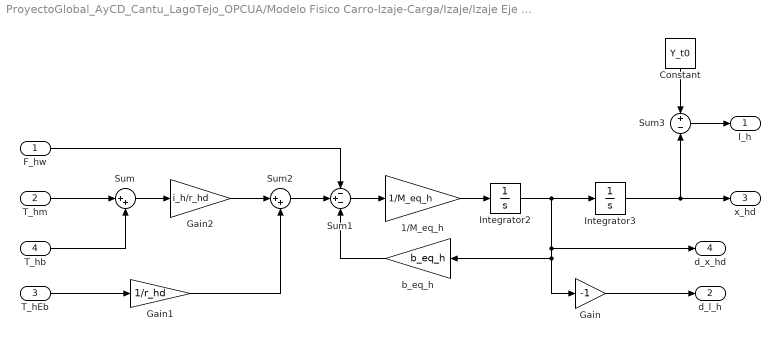
== system ProyectoGlobal_AyCD_Cantu_LagoTejo_OPCUA/Modelo Fisico Carro-Izaje-Carga/Izaje/Izaje Eje Rapido-Lento ==
  F_hw : Inport
  T_hm : Inport  Port=2
  T_hEb : Inport  Port=3
  T_hb : Inport  Port=4
  1/M_eq_h : Gain  Gain=1/M_eq_h
  Constant : Constant  Value=Y_t0
  Gain : Gain  Gain=-1
  Gain1 : Gain  Gain=1/r_hd
  Gain2 : Gain  Gain=i_h/r_hd
  Integrator2 : Integrator
  Integrator3 : Integrator  InitialCondition=CI_h
  Sum : Sum  Inputs=|++
  Sum1 : Sum  Inputs=-+-
  Sum2 : Sum  Inputs=|++
  Sum3 : Sum  Inputs=+|-
  b_eq_h : Gain  Gain=b_eq_h
  l_h : Outport
  d_l_h : Outport  Port=2
  x_hd : Outport  Port=3
  d_x_hd : Outport  Port=4
  wires:
  Integrator2/1 -> Gain/1, b_eq_h/1, d_x_hd/1, Integrator3/1
  1/M_eq_h/1 -> Integrator2/1
  b_eq_h/1 -> Sum1/3
  F_hw/1 -> Sum1/1
  T_hm/1 -> Sum/1
  T_hEb/1 -> Gain1/1
  T_hb/1 -> Sum/2
  Constant/1 -> Sum3/1
  Sum3/1 -> l_h/1
  Integrator3/1 -> x_hd/1, Sum3/2
  Sum1/1 -> 1/M_eq_h/1
  Sum/1 -> Gain2/1
  Gain/1 -> d_l_h/1
  Sum2/1 -> Sum1/2
  Gain1/1 -> Sum2/2
  Gain2/1 -> Sum2/1

== system ProyectoGlobal_AyCD_Cantu_LagoTejo_OPCUA/Modelo Fisico Carro-Izaje-Carga/Limites de operacion/Límites de Carro ==
  x_t : Inport
  Constant : Constant  Value=lim_xIzq_ult
  Constant1 : Constant  Value=lim_xIzq
  Constant2 : Constant  Value=lim_xDer_ult
  Constant3 : Constant  Value=lim_xDer
  Equal : RelationalOperator  Operator=<=  OutDataTypeStr=boolean  RndMeth=Simplest
  Equal1 : RelationalOperator  Operator=<=  OutDataTypeStr=boolean  RndMeth=Simplest
  Equal2 : RelationalOperator  OutDataTypeStr=boolean  RndMeth=Simplest
  Equal3 : RelationalOperator  OutDataTypeStr=boolean  RndMeth=Simplest
  fc_izq_norm : Outport
  fc_izq_ult : Outport  Port=2
  fc_der_norm : Outport  Port=3
  fc_der_ult : Outport  Port=4
  wires:
  Constant/1 -> Equal1/2
  Constant1/1 -> Equal/2
  Constant3/1 -> Equal2/2
  Constant2/1 -> Equal3/2
  Equal1/1 -> fc_izq_ult/1
  Equal3/1 -> fc_der_ult/1
  Equal2/1 -> fc_der_norm/1
  x_t/1 -> Equal2/1, Equal3/1, Equal1/1, Equal/1
  Equal/1 -> fc_izq_norm/1

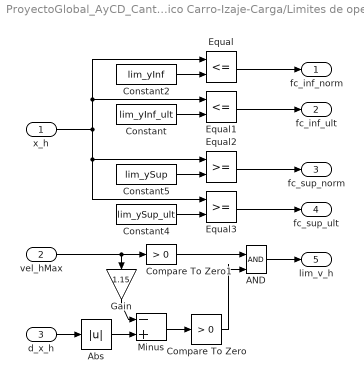
== system ProyectoGlobal_AyCD_Cantu_LagoTejo_OPCUA/Modelo Fisico Carro-Izaje-Carga/Limites de operacion/Subsystem1 ==
  x_h : Inport
  vel_hMax : Inport  Port=2
  d_x_h : Inport  Port=3
  AND : Logic  IconShape=distinctive  AllPortsSameDT=off  OutDataTypeStr=boolean
  Abs : Abs
  Compare To Zero : simulink/Logic and Bit Operations/Compare To Zero  relop=>  OutDataTypeStr=boolean
  Compare To Zero1 : simulink/Logic and Bit Operations/Compare To Zero  relop=>  OutDataTypeStr=boolean
  Constant : Constant  Value=lim_yInf_ult
  Constant2 : Constant  Value=lim_yInf
  Constant4 : Constant  Value=lim_ySup_ult
  Constant5 : Constant  Value=lim_ySup
  Equal : RelationalOperator  Operator=<=  OutDataTypeStr=boolean  RndMeth=Simplest
  Equal1 : RelationalOperator  Operator=<=  OutDataTypeStr=boolean  RndMeth=Simplest
  Equal2 : RelationalOperator  OutDataTypeStr=boolean  RndMeth=Simplest
  Equal3 : RelationalOperator  OutDataTypeStr=boolean  RndMeth=Simplest
  Gain : Gain  Gain=1.15
  Minus : Sum  Inputs=-+
  fc_inf_norm : Outport
  fc_inf_ult : Outport  Port=2
  fc_sup_norm : Outport  Port=3
  fc_sup_ult : Outport  Port=4
  lim_v_h : Outport  Port=5
  wires:
  Abs/1 -> Minus/2
  vel_hMax/1 -> Gain/1, Compare To Zero1/1
  d_x_h/1 -> Abs/1
  Minus/1 -> Compare To Zero/1
  Constant4/1 -> Equal3/2
  Equal1/1 -> fc_inf_ult/1
  Equal/1 -> fc_inf_norm/1
  Constant/1 -> Equal1/2
  Equal3/1 -> fc_sup_ult/1
  Constant5/1 -> Equal2/2
  Equal2/1 -> fc_sup_norm/1
  x_h/1 -> Equal2/1, Equal3/1, Equal1/1, Equal/1
  Constant2/1 -> Equal/2
  AND/1 -> lim_v_h/1
  Compare To Zero1/1 -> AND/1
  Compare To Zero/1 -> AND/2
  Gain/1 -> Minus/1

== system ProyectoGlobal_AyCD_Cantu_LagoTejo_OPCUA/Modelo Fisico Carro-Izaje-Carga/theta y l/Subsystem ==
  x_l : Inport
  d_x_l : Inport  Port=2
  x_t : Inport  Port=3
  d_x_t : Inport  Port=4
  y_l : Inport  Port=5
  d_y_l : Inport  Port=6
  l : Inport  Port=7
  Constant : Constant  Value=Y_t0
  Divide : Product  Inputs=*/
  Product : Product
  Product1 : Product
  Sum{,1..3} (4 alike) : Sum  Inputs=+|-
  d_l : Outport
  wires:
  l/1 -> Divide/2
  Product/1 -> Sum/1
  Product1/1 -> Sum/2
  x_l/1 -> Sum1/1
  x_t/1 -> Sum1/2
  Sum1/1 -> Product/1
  d_x_l/1 -> Sum2/1
  d_x_t/1 -> Sum2/2
  Sum2/1 -> Product/2
  d_y_l/1 -> Product1/1
  Constant/1 -> Sum3/1
  y_l/1 -> Sum3/2
  Sum3/1 -> Product1/2
  Sum/1 -> Divide/1
  Divide/1 -> d_l/1

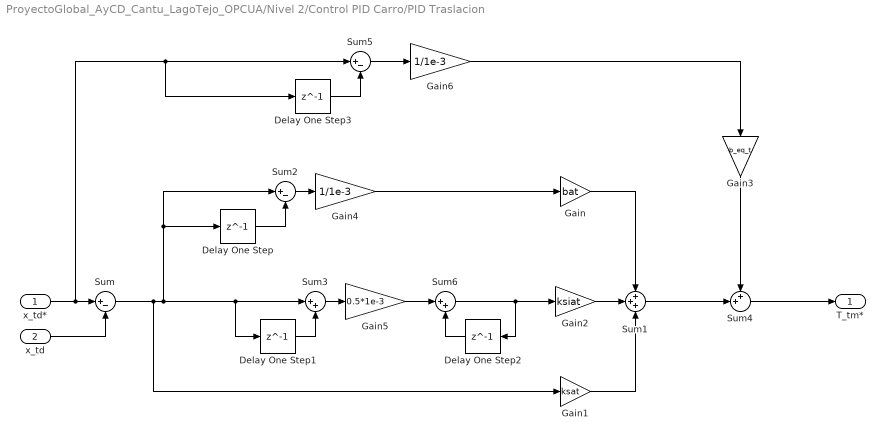
== system ProyectoGlobal_AyCD_Cantu_LagoTejo_OPCUA/Nivel 2/Control PID Carro/PID Traslacion ==
  x_td* : Inport
  x_td : Inport  Port=2
  Delay One Step{,1..3} (4 alike) : Delay  DelayLength=1  SampleTime=1e-3
  Gain : Gain  Gain=bat
  Gain1 : Gain  Gain=ksat
  Gain2 : Gain  Gain=ksiat
  Gain3 : Gain  Gain=b_eq_t
  Gain4 : Gain  Gain=1/1e-3
  Gain5 : Gain  Gain=0.5*1e-3
  Gain6 : Gain  Gain=1/1e-3
  Sum : Sum  Inputs=|+-
  Sum1 : Sum  Inputs=+++
  Sum2 : Sum  Inputs=|+-
  Sum3 : Sum  Inputs=|++
  Sum4 : Sum  Inputs=++|
  Sum5 : Sum  Inputs=|+-
  Sum6 : Sum  Inputs=|++
  T_tm* : Outport
  wires:
  x_td/1 -> Sum/2
  Gain/1 -> Sum1/1
  Gain1/1 -> Sum1/3
  Gain2/1 -> Sum1/2
  Sum/1 -> Delay One Step/1, Sum2/1, Delay One Step1/1, Sum3/1, Gain1/1
  Gain4/1 -> Gain/1
  Gain3/1 -> Sum4/1
  Sum1/1 -> Sum4/2
  Sum4/1 -> T_tm*/1
  Sum2/1 -> Gain4/1
  Delay One Step/1 -> Sum2/2
  Sum3/1 -> Gain5/1
  Delay One Step1/1 -> Sum3/2
  Sum5/1 -> Gain6/1
  Delay One Step3/1 -> Sum5/2
  x_td*/1 -> Delay One Step3/1, Sum5/1, Sum/1
  Gain6/1 -> Gain3/1
  Gain5/1 -> Sum6/1
  Sum6/1 -> Delay One Step2/1, Gain2/1
  Delay One Step2/1 -> Sum6/2

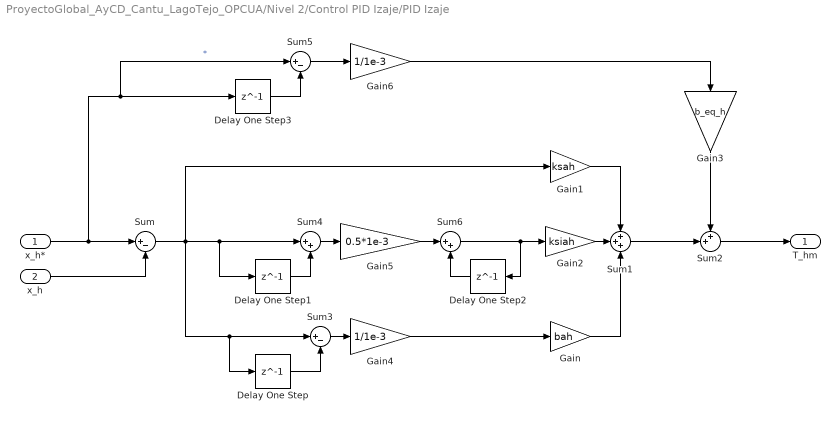
== system ProyectoGlobal_AyCD_Cantu_LagoTejo_OPCUA/Nivel 2/Control PID Izaje/PID Izaje ==
  x_h* : Inport
  x_h : Inport  Port=2
  Delay One Step{,1..3} (4 alike) : Delay  DelayLength=1  SampleTime=1e-3
  Gain : Gain  Gain=bah
  Gain1 : Gain  Gain=ksah
  Gain2 : Gain  Gain=ksiah
  Gain3 : Gain  Gain=b_eq_h
  Gain4 : Gain  Gain=1/1e-3
  Gain5 : Gain  Gain=0.5*1e-3
  Gain6 : Gain  Gain=1/1e-3
  Sum : Sum  Inputs=|+-
  Sum1 : Sum  Inputs=+++
  Sum2 : Sum  Inputs=++|
  Sum3 : Sum  Inputs=|+-
  Sum4 : Sum  Inputs=|++
  Sum5 : Sum  Inputs=|+-
  Sum6 : Sum  Inputs=|++
  T_hm : Outport
  wires:
  Gain2/1 -> Sum1/2
  Gain1/1 -> Sum1/1
  Gain/1 -> Sum1/3
  x_h/1 -> Sum/2
  Gain3/1 -> Sum2/1
  Sum1/1 -> Sum2/2
  Sum2/1 -> T_hm/1
  Sum3/1 -> Gain4/1
  Gain4/1 -> Gain/1
  Delay One Step/1 -> Sum3/2
  Sum4/1 -> Gain5/1
  Delay One Step1/1 -> Sum4/2
  Sum/1 -> Delay One Step1/1, Sum4/1, Delay One Step/1, Sum3/1, Gain1/1
  Sum6/1 -> Gain2/1, Delay One Step2/1
  Gain6/1 -> Gain3/1
  Delay One Step3/1 -> Sum5/2
  Sum5/1 -> Gain6/1
  Delay One Step2/1 -> Sum6/2
  Gain5/1 -> Sum6/1
  x_h*/1 -> Sum/1, Sum5/1, Delay One Step3/1  "*"

== system ProyectoGlobal_AyCD_Cantu_LagoTejo_OPCUA/Modelo Fisico Carro-Izaje-Carga/Izaje/Fuerza cable de Izaje/K_w ==
  l_h : Inport
  Constant3 : Constant  Value=k_wu
  Constant4 : Constant  Value=110
  Divide2 : Product  Inputs=*/
  Gain6 : Gain  Gain=2
  Sum2 : Sum  Inputs=|++
  K_w : Outport
  wires:
  Sum2/1 -> Divide2/2
  Gain6/1 -> Sum2/1
  Constant3/1 -> Divide2/1
  Constant4/1 -> Sum2/2
  Divide2/1 -> K_w/1
  l_h/1 -> Gain6/1

== system ProyectoGlobal_AyCD_Cantu_LagoTejo_OPCUA/Modelo Fisico Carro-Izaje-Carga/Izaje/Fuerza cable de Izaje/b_w ==
  l_h : Inport
  Constant3 : Constant  Value=b_wu
  Constant4 : Constant  Value=110
  Gain6 : Gain  Gain=2
  Product : Product
  Sum2 : Sum  Inputs=|++
  b_w : Outport
  wires:
  Sum2/1 -> Product/2
  Gain6/1 -> Sum2/1
  Constant3/1 -> Product/1
  Constant4/1 -> Sum2/2
  Product/1 -> b_w/1
  l_h/1 -> Gain6/1

== matlab function ProyectoGlobal_AyCD_Cantu_LagoTejo_OPCUA/Modelo Fisico Carro-Izaje-Carga/Modos de Contacto/MATLAB Function1 ==
  data: Susp input; Y_c0 output size=1; x_l input; Yc input; Xc input; TLK input; TLKold input; yc_act_old input size=[1 32]; yc_act output size=[1 32]; change output size=1
function [Y_c0,yc_act,  change] = yc_actual(Susp,x_l,Yc,Xc,TLK,TLKold,yc_act_old)
%Susp: modo de contacto (1 suspendido , 0 apoyado)
change=0;

%yc_act = zeros(1,length(yc));
%Posicionamiento de container en el plano
idx=1;

for i=1:length(Xc)
    if ((x_l>=(Xc(i)-1.25))&&(x_l<(Xc(i)+1.25)))
        idx = i;
    end
end

if(yc_act_old == Yc)
    %Cierra el Twistlock -> Container tomado(Se quita del suelo)
    if((TLK==1) && (TLKold==0) && (Susp==0))
        
        if(x_l>2.5 && x_l<47.5)
            
            if(Yc(idx)>-20 )
                Yc(idx) = Yc(idx) - 2.5;
            end
            yc_act = Yc;
            Y_c0 = yc_act(idx);
            change=1;
            
        elseif(x_l>-37.5 && x_l <-2.5)
            
            if(Yc(idx)>0)
                Yc(idx) = Yc(idx) - 2.5;
            end
            yc_act = Yc;
            Y_c0 = yc_act(idx);
            change=1;
            
        end
        
        %Abre el Twistlock -> Container posicionado y soltado(Se agrega al suelo)
    elseif((TLK==0) && (TLKold==1) && (Susp==0))
        if(Yc(idx)<32.5 )
            Yc(idx) = Yc(idx) + 2.5;
        end
        yc_act = Yc;
        Y_c0 = yc_act(idx);
        change=1;
    else
        change=0;
    end
    
end




yc_act = Yc;
Y_c0 = yc_act(idx);
end

== matlab function ProyectoGlobal_AyCD_Cantu_LagoTejo_OPCUA/Nivel 2/MATLAB Function ==
  data: m_l input; l_h input; Kp output; Kd output; kd_bal input; kp_bal input
function [Kp,Kd] = fcn(m_l,l_h,kd_bal,kp_bal)
index_ml = ceil(m_l/100);
index_h = ceil(l_h/0.1);
if(index_ml <= 1)
   index_ml = 1; 
end

if(index_h <= 1)
   index_h = 1; 
end

if(index_ml >= 51)
   index_ml = 51; 
end

if(index_h >= 60)
   index_h = 60; 
end
Kd = kd_bal(index_ml,index_h);
Kp = kp_bal(index_ml,index_h);

end

== stateflow chart ProyectoGlobal_AyCD_Cantu_LagoTejo_OPCUA/Modelo Fisico Carro-Izaje-Carga/Chart ==
  settings: sampleTime=1e-3
  state CONTENEDOR_REAL [parallel]
    settings: executionOrder=1
    state CARGADO
      entry:
      h_c=H_c;
      M_cX = randi(M_cMax - M_cMin)+M_cMin;
      m_l_real=M_s+M_cX;
      %Ow = 10000;
      %Mc_min = 2000;
      %Mc_max = 50000;
      %mRand = randi([Mc_min Mc_max+Ow],1);
      %ml_asignada=Ms+mRand;
      %ml_asignada=75000;
      %ml_asignada=65000; %CARGA MAX
      %ml_asignada=40000; % MEDIA CARGA
    state DESCARGADO
      entry:
      m_l_real=M_s;
      h_c=0;
    (default) -> DESCARGADO
    CARGADO -> DESCARGADO : [cargado == 0]
    DESCARGADO -> CARGADO : [cargado == 1]
  state GRAFICA_PERFIL [parallel]
    entry:
    x_trm_plot=0;
    graficar=1;
    x_c=xc;
    y_c=yc;
    during:
    x_trm_plot=x_trm_plot+1e-3;
    if(change==1)
    y_c=yc_act;
    end
    if((x_trm_plot>0.998)&&(x_trm_plot<1.002))
    graficar=1;
    x_trm_plot=0;
    else
    graficar=0;
    end
    settings: executionOrder=2
  data: cargado input; M_s parameter; Mc_max local double size=1; Ow local double size=1; Mc_min local double size=1; mRand local double size=1; h_c output double size=1; H_c parameter; x_aux local double size=[1 40]; y_c output size=[1 32]; change input; yc_act input size=[1 32]; graficar output size=1; x_trm_plot local; i local; yc2 local double; x_c output; xc parameter; yc parameter; M_cMin parameter; M_cMax parameter; M_cX local double size=1; m_l_real output

== matlab function ProyectoGlobal_AyCD_Cantu_LagoTejo_OPCUA/MATLAB Function1 ==
  data: clock input; ON_OFF input; BTN_EMERGENCIA input; Manual input; Ciclo input; max_masa input; Tension_hw input; lim_v_h input; Balanceo input; manual_auto input; ml_medida input; xc input; yc input; graficar input; x_l input; y_l input; x_td input
function grafico_puerto(clock, ON_OFF, BTN_EMERGENCIA, Manual, Ciclo, max_masa, Tension_hw, lim_v_h, Balanceo, manual_auto, ml_medida, xc, yc, graficar, x_l, y_l, x_td)
if(graficar==1)
    alt_txt = 14;   color_cont = "#90AC50";
    fh = figure(100);
    %fh.WindowState = 'maximized';
    clf(fh);
    %figure(100);
    title('Simulación Visual en Tiempo "Real"'),    grid on
    rectangle('Position',[-30, 46, 80, 4],'FaceColor', '#EEEEEE','EdgeColor','#EEEEEE')
    rectangle('Position',[-30, -20, 30, 20],'FaceColor', 'w')
    line([-30 0],[-0.5 -0.5],'Color','black','LineWidth', 5)                    %%% Muelle
    rectangle('Position',[-0.5, 0, 0.5, 15],'FaceColor','black');               %%% Sill Beam
    rectangle('Position',[0.5, -20, 49.5, 25],'EdgeColor','b','LineWidth', 1.5);%%% Barco
    rectangle('Position',[-30, 45, 80, 2],'FaceColor',[0.8 0.8 1]);             %%% Grúa
    rectangle('Position',[x_l-1.25,y_l,2.5,0.5],'FaceColor','k');               %%% Spreader
    rectangle('Position',[x_td-2.5, 45, 5, 2],'FaceColor','k');              %%% Carro
    line([x_l x_td], [y_l 45],'Color','black','LineWidth',2)                 %%% Cable

    for i=1:length(yc)                  %%% Perfil de Carga
        if (xc(i)<2.5)                  %%% Lado de Muelle
            rectangle('Position',[xc(i)-1.25,0,2.5,yc(i)],'FaceColor', color_cont,'LineWidth', 0.3);
        elseif(xc(i)>2.5 && xc(i)<47.5) %%% Lado de Barco
            rectangle('Position',[xc(i)-1.25,-20,2.5,yc(i)+20],'FaceColor', color_cont,'LineWidth', 0.3);
        end
    end

    txt000 = {'Tiempo: ', clock};       %%% Tiempo de Ejecución "Real"
    text(-10, -3.5, txt000,'FontSize', alt_txt)

    if(ON_OFF)                          %%% Cartel de ON - OFF
        txt00 = {'ON: Encendido'};
        text(-30,48.5,txt00,'FontSize',alt_txt,'Color',"#00AA00")
    else
        txt00 = {'OFF: APAGADO'};
        text(-30,48.5,txt00,'FontSize',alt_txt,'Color',"#FF0000")
    end
    
    txt = {'Masa: ', ml_medida};               %%% Cartel de Masa Total en Spreader
    text(-29.75,-17,txt,'FontSize',alt_txt)

    if (ml_medida > 15000)                       %%% Cartel de Cargado/Sin Carga/SOBRECARGA
        rectangle('Position',[x_l-1.25,y_l-2.5,2.5,2.5],'FaceColor', color_cont,'LineWidth', 0.3); %carga
        if (max_masa)
            txt01 = {'SOBRECARGA'};
            text(-25,-17,txt01,'Color','red','FontSize',alt_txt+2)
        else
            txt01 = {'Cargado'};
            text(-25,-17,txt01,'Color',"#00AA00",'FontSize',alt_txt)
        end
    else
        txt01 = {'Sin Carga'};
        text(-25,-17,txt01,'Color',"#CB7A00",'FontSize',alt_txt)
    end

    if (Manual)                       %%% Cartel de Modo de Control
        txt02 = {'Manual'};
        text(-15, 48.5,txt02,'FontSize', alt_txt)
    else
        if (manual_auto)
            txt02 = {'Automático'};
            text(-15, 48.5,txt02,'FontSize',alt_txt)
        else
            txt02 = {'Manual'};
            text(-15, 48.5,txt02,'FontSize',alt_txt)
        end
    end

    if (Balanceo)                       %%% Cartel de Control de Balanceo
        txt03 = {'Balanceo: ON'};
        text(-4, 48.5, txt03,'FontSize',alt_txt,'Color',"#00AA00")
    else
        txt03 = {'Balanceo: OFF'};
        text(-4, 48.5,txt03,'FontSize', alt_txt,'Color','#FF0000')
    end

    if (Tension_hw)                     %%% Cartel de Spreader Apoyado o Suspendido
        txt04 = {'Suspendido'};
        text(10,48.5,txt04,'FontSize', alt_txt)
    else
        txt04 = {'Apoyado'};
        text(10,48.5,txt04,'FontSize', alt_txt)
    end

    if (Ciclo)                          %%% Cartel de Tipo de Ciclo
        txt05 = {'Ciclo Doble'};
        text(22,48.5,txt05,'FontSize', alt_txt)
    else
        txt05 = {'Ciclo Simple'};
        text(22,48.5,txt05,'FontSize', alt_txt)
    end
    
    if (BTN_EMERGENCIA)                 %%% Cartel de EMERGENCIA (botón)
        txt7 = {'EMERGENCIA'};
        rectangle('Position',[34.5, 47, 15.5, 3],'FaceColor', 'red')
        text(35.5,48.5,txt7,'FontSize', alt_txt+6,'Color',"w")
    else
        txt7 = {'OK'};
        rectangle('Position',[34.5, 47, 15.5, 3],'FaceColor', "#00FF00")
        text(41,48.5,txt7,'FontSize', alt_txt+6,'Color',"k")
    end
  
    txt1 = {'Carro (X): ',x_td};                %%% Posiciones del Carro
    text(-29.75,-3.5,txt1,'FontSize',alt_txt)
    txt1 = {'Carro (Y): ',45};
    text(-20,-3.5,txt1,'FontSize',alt_txt)
    txt1 = {'Spreader (X): ',x_l};              %%% Posiciones del Spreader
    text(-29.75,-10,txt1,'FontSize',alt_txt)
    txt1 = {'Spreader (Y): ',y_l};
    text(-20,-10,txt1,'FontSize',alt_txt)
end
end

== matlab function ProyectoGlobal_AyCD_Cantu_LagoTejo_OPCUA/MATLAB Function ==
  data: carrilFin input; X_fin output; carrilFinDoble input; Xcarga input; X_finDoble output
function [X_fin, X_finDoble] = carril2x(carrilFin, carrilFinDoble, Xcarga)
offsetCarrilesBarco = 13; % Total carriles:32 - carriles en barco:18 - carril final:1 =13

X_fin = Xcarga(carrilFin + offsetCarrilesBarco);
X_finDoble = Xcarga(carrilFinDoble + offsetCarrilesBarco);
end

== matlab function ProyectoGlobal_AyCD_Cantu_LagoTejo_OPCUA/Modelo Fisico Carro-Izaje-Carga/Modos de Contacto/MATLAB Function2 ==
  data: Susp input; Y_c0 output; x_l input; yc_act output; yc input; TLK input; TLK_ant input; change output; yc_act_ant input
function [Y_c0,yc_act,change] = update_yc(Susp,x_l,yc,TLK,TLK_ant,yc_act_ant)
%Susp -> modo de contacto (1 suspendido , 0 apoyado)
change=0;

%Posicionamiento de container en el plano
idx=1;
for i=1:length(yc(1,:))
    if ((x_l>=(yc(1,i)-1.25))&&(x_l<(yc(1,i)+1.25)))
        idx = i;
    end
end


if(yc_act_ant == yc)
    %Cierra el Twistlock -> Container tomado(Se quita del suelo)
    if((TLK==1) && (TLK_ant==0) && (Susp==0))

        if(x_l>2.5 && x_l <47.5)   

            if(yc(2,idx)>-20 )
                yc(2,idx) = yc(2,idx) - 2.5;
            end
            yc_act = yc;
            Y_c0 = yc_act(2,idx);
            change=1;

        elseif(x_l>-37.5 && x_l <-2.5)

            if(yc(2,idx)>0 )
                yc(2,idx) = yc(2,idx) - 2.5;
            end
            yc_act = yc;
            Y_c0 = yc_act(2,idx);
            change=1;

        end

    %Abre el Twistlock -> Container posicionado y soltado(Se agrega al suelo)
    elseif((TLK==0) && (TLK_ant==1) && (Susp==0))
        if(yc(2,idx)<32.5 )
            yc(2,idx) = yc(2,idx) + 2.5;        
        end
        yc_act = yc;
        Y_c0 = yc_act(2,idx);
        change=1;
    else
        change=0;
    end
    
end

yc_act = yc;
Y_c0 = yc_act(2,idx);

end
